simulink model "vehicle_6dof_model"  (R2025b)
settings: Solver=VariableStepAuto  StartTime=0.0  StopTime=10.0  RelTol=1e-3
model workspace (MAT data in the model file):
  mmoi = [0.01211163  -3.59e-06  1.486e-05; -3.59e-06  0.01211098  -4.75e-07; 1.486e-05  -4.75e-07  0.00012254]
libraries: aerolibanim x1, aerolibanimutils x1
settings Model: Creator=Josh Fernandez  LastModifiedBy=Josh

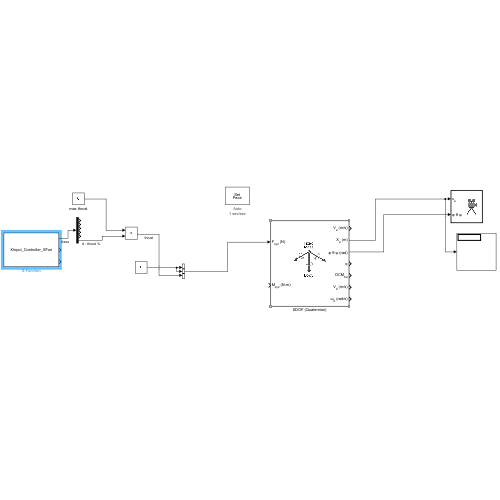
[thumbnail: Simulink's stored preview of the top-level diagram]
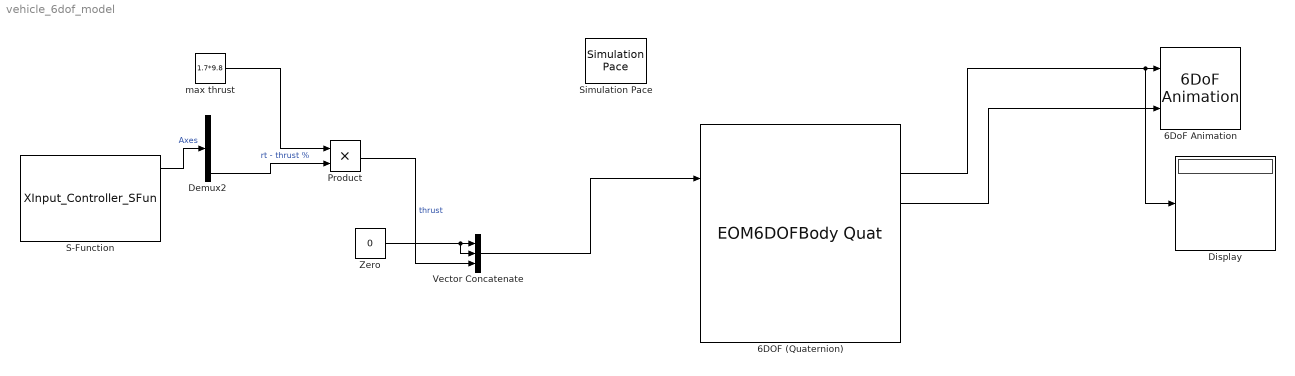
== system vehicle_6dof_model ==
  6DOF (Quaternion) : EOM6DOFBodyQuat  mass_0=.5384  inertia=mmoi
  6DoF Animation : aerolibanim/6DoF Animation  u1=[0 4000 -2000 2000 -5000 -3000]  u2=0.1  u3=1.0  u4=[4000 0 -5000]  u5=Fixed position  u6=[2000 500 -3150]  u7=10  u8=on
  Demux2 : Demux  Outputs=6
  Display : Display
  Product : Product
  S-Function : S-Function  FunctionName=XInput_Controller_SFun  Parameters=1  SFunctionDeploymentMode=off  EnableBusSupport=off
  Simulation Pace : aerolibanimutils/Simulation Pace  SimulationPace=1  SleepMode=Auto  OutputPaceError=off  SampleTime=1/30
  Vector Concatenate : Concatenate  NumInputs=3
  Zero : Constant  Value=0  OutDataTypeStr=Inherit: Inherit via back propagation
  max thrust : Constant  Value=1.7*9.8
  wires:
  6DOF (Quaternion)/2 -> Display/1, 6DoF Animation/1
  6DOF (Quaternion)/3 -> 6DoF Animation/2
  S-Function/1 -> Demux2/1  "Axes"
  Demux2/6 -> Product/2  "rt - thrust %"
  max thrust/1 -> Product/1
  Product/1 -> Vector Concatenate/3  "thrust"
  Zero/1 -> Vector Concatenate/2, Vector Concatenate/1
  Vector Concatenate/1 -> 6DOF (Quaternion)/1
